simulink model "LQG_sim_lin_kalman"  (R2016b)
settings: Solver=VariableStepAuto  StartTime=0.0  StopTime=60  FixedStep=Ts  RelTol=1e-3
values from neighbouring files (symbols this model uses):
  A_0 = [0 -3.26931291643 0 0.71460251427 0 0 0 0 1 -0.0325743287495 0 -0.000548520916999 ... (64 elements, 8x8)]    [parametros.mat]    (also in twin_rotor_modelo_V1.m = eval(A_0))
  B_0 = [0 0 0 0 0 0 1190.47619048 0 0 0 0 0 ... (16 elements, 8x2)]    [parametros.mat]    (also in twin_rotor_modelo_V1.m = eval(B_0))
  C_0 = [1 0 0 0 0 1 0 0 0 0 0 0 ... (16 elements, 2x8)]    [parametros.mat]    (also in twin_rotor_modelo_V1.m = eval(C_0))
  ci = zeros(1,8)    [LQR.m]    (also in MIMO.m)
  D_0 = [0  0; 0  0]    [parametros.mat]    (also in twin_rotor_modelo_V1.m = eval(D_0))
  L = Ec-Ep    [twin_rotor_modelo_V1.m]
undefined symbols (not defined in the file or in its folder): K
settings Model: Creator=cristobal  LastModifiedBy=cristobal

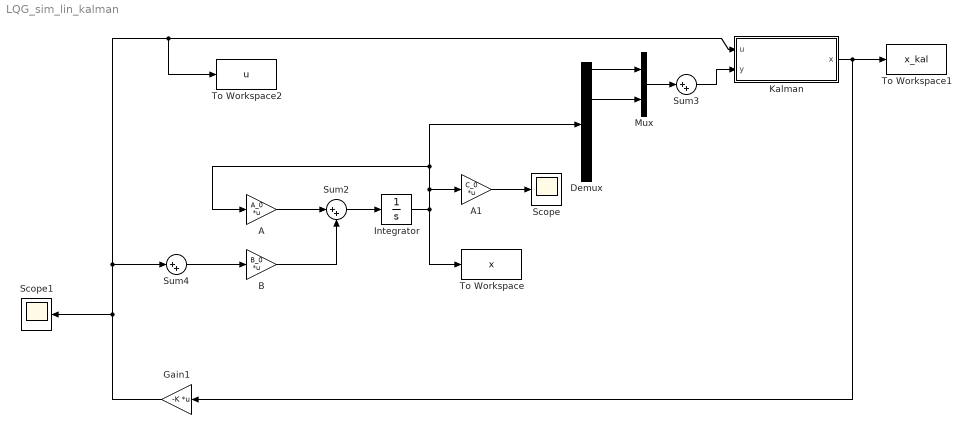
== system LQG_sim_lin_kalman ==
  A : Gain  Gain=A_0  Multiplication=Matrix(K*u)
  A1 : Gain  Gain=C_0  Multiplication=Matrix(K*u)
  B : Gain  Gain=B_0  Multiplication=Matrix(K*u)
  Demux : Demux  Outputs=8
  Gain1 : Gain  Gain=-K  Multiplication=Matrix(K*u)
  Integrator : Integrator  InitialCondition=ci
  Kalman : Subsystem
  Mux : Mux  Inputs=2
  Scope : Scope
  Scope1 : Scope
  Sum2 : Sum  Inputs=|++
  Sum3 : Sum  Inputs=|++
  Sum4 : Sum  Inputs=|++
  To Workspace : ToWorkspace  VariableName=x  SaveFormat=Timeseries  SampleTime=-1
  To Workspace1 : ToWorkspace  VariableName=x_kal  SaveFormat=Timeseries  SampleTime=-1
  To Workspace2 : ToWorkspace  VariableName=u  SaveFormat=Timeseries  SampleTime=-1
  wires:
  Integrator/1 -> A1/1, Demux/1, A/1, To Workspace/1
  A/1 -> Sum2/1
  B/1 -> Sum2/2
  Sum2/1 -> Integrator/1
  Gain1/1 -> Scope1/1, Sum4/1, To Workspace2/1, Kalman/1(u)
  A1/1 -> Scope/1
  Demux/1 -> Mux/1
  Demux/3 -> Mux/2
  Kalman/1(x) -> Gain1/1, To Workspace1/1
  Mux/1 -> Sum3/1
  Sum3/1 -> Kalman/2(y)
  Sum4/1 -> B/1

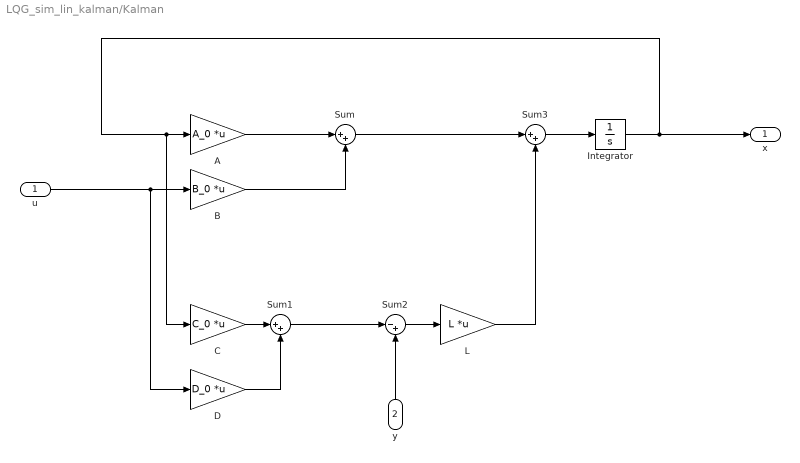
== system LQG_sim_lin_kalman/Kalman ==
  u : Inport
  y : Inport  Port=2
  A : Gain  Gain=A_0  Multiplication=Matrix(K*u)
  B : Gain  Gain=B_0  Multiplication=Matrix(K*u)
  C : Gain  Gain=C_0  Multiplication=Matrix(K*u)
  D : Gain  Gain=D_0  Multiplication=Matrix(K*u)
  Integrator : Integrator
  L : Gain  Gain=L  Multiplication=Matrix(K*u)
  Sum : Sum  Inputs=|++
  Sum1 : Sum  Inputs=|++
  Sum2 : Sum  Inputs=|-+
  Sum3 : Sum  Inputs=|++
  x : Outport
  wires:
  Integrator/1 -> C/1, A/1, x/1
  u/1 -> D/1, B/1
  A/1 -> Sum/1
  B/1 -> Sum/2
  C/1 -> Sum1/1
  D/1 -> Sum1/2
  y/1 -> Sum2/2
  Sum1/1 -> Sum2/1
  Sum2/1 -> L/1
  Sum/1 -> Sum3/1
  L/1 -> Sum3/2
  Sum3/1 -> Integrator/1
